simulink model "Steam_Turbine"  (R2024b)
settings: Solver=VariableStepAuto  StartTime=0.0  StopTime=50  RelTol=1e-3
settings Model: Creator=HP  LastModifiedBy=HP

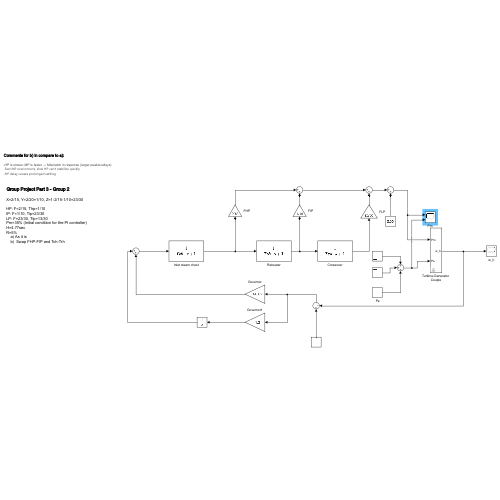
[thumbnail: Simulink's stored preview of the top-level diagram]
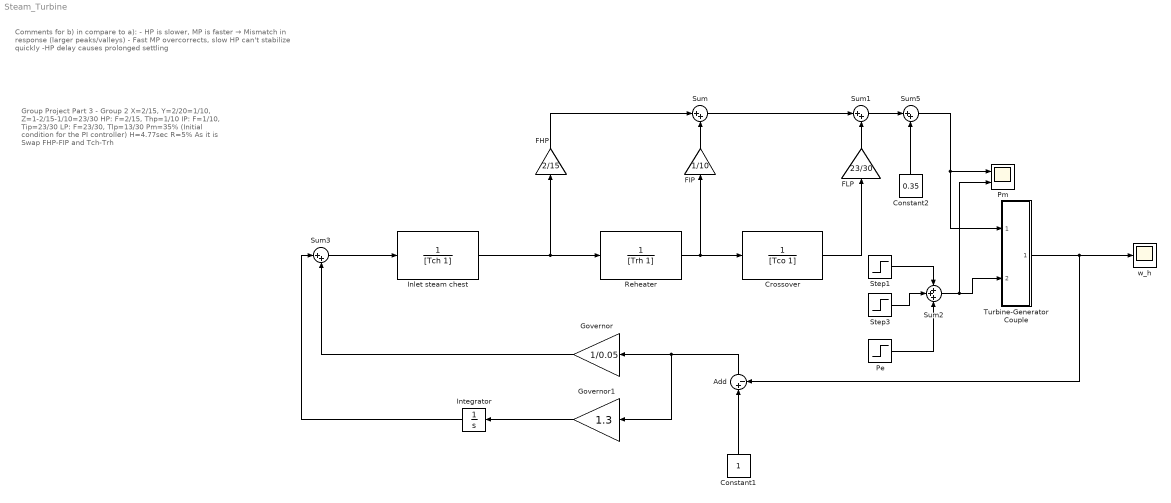
== system Steam_Turbine ==
  note: Comments for b) in compare to a):
      |
      | - HP is slower, MP is faster → Mismatch in response (larger peaks/valleys)
      | - Fast MP overcorrects, slow HP can't stabilize quickly
      | -HP delay causes prolonged settling
  note: Group Project Part 3 - Group 2
      |
      | X=2/15, Y=2/20=1/10, Z=1-2/15-1/10=23/30
      |
      | HP: F=2/15, Thp=1/10
      | IP: F=1/10, Tip=23/30
      | LP: F=23/30, Tlp=13/30
      | Pm=35% (Initial condition for the PI controller)
      | H=4.77sec
      | R=5%
      | As it is
      | Swap FHP-FIP and Tch-Trh
  " Pe" : Step  Time=15  Before=0.15  After=0.45  SampleTime=0
  Add : Sum  Inputs=|+-
  Constant1 : Constant
  Constant2 : Constant  Value=0.35
  Crossover : TransferFcn  Denominator=[Tco 1]  mask{Tco=13/30}
      mask prompts: Tco "Crossover Time Constant / Low-Pressure (LP) Turbine Time Constant)"
      mask DialogControl ParameterGroupVar Prompt: Parameters
  FHP : Gain  Gain=2/15
  FIP : Gain  Gain=1/10
  FLP : Gain  Gain=23/30
  Governor : Gain  Gain=1/0.05
  Governor1 : Gain  Gain=1.3
  Inlet steam chest : TransferFcn  Denominator=[Tch 1]  mask{Tch=1/10}
      mask prompts: Tch "HP cynlinder time constant"
      mask DialogControl ParameterGroupVar Prompt: Parameters
  Integrator : Integrator
  Pm : Scope  NumInputPorts=2
  Reheater : TransferFcn  Denominator=[Trh 1]  mask{Trh=23/30}
      mask prompts: Trh "Reheater Time Constant"
      mask DialogControl ParameterGroupVar Prompt: Parameters
  Step1 : Step  Time=5  Before=0.10  After=0.35  SampleTime=0
  Step3 : Step  Time=10  Before=0.10  After=-0.30  SampleTime=0
  Sum{,1,3,5} (4 alike) : Sum  Inputs=|++
  Sum2 : Sum  Inputs=+++
  Turbine-Generator Couple : Subsystem  mask{Hh=4.77, w_ini=1}
      mask prompts: Hh "H/E Inertia Constant"; w_ini "Initial omega"
  w_h : Scope
  wires:
  Sum5/1 -> Turbine-Generator Couple/1(Pm), Pm/1
  Inlet steam chest/1 -> FHP/1, Reheater/1
  FHP/1 -> Sum/1
  Sum/1 -> Sum1/1
  FLP/1 -> Sum1/2
  FIP/1 -> Sum/2
  Turbine-Generator Couple/1(w_h) -> Add/2, w_h/1
  Constant1/1 -> Add/1
  Add/1 -> Governor1/1, Governor/1
  Reheater/1 -> Crossover/1, FIP/1
  Crossover/1 -> FLP/1
  Governor1/1 -> Integrator/1
  Integrator/1 -> Sum3/1
  Governor/1 -> Sum3/2
  Sum3/1 -> Inlet steam chest/1
  Step1/1 -> Sum2/1
  " Pe"/1 -> Sum2/3
  Step3/1 -> Sum2/2
  Sum2/1 -> Pm/2, Turbine-Generator Couple/2(Pe)
  Sum1/1 -> Sum5/1
  Constant2/1 -> Sum5/2

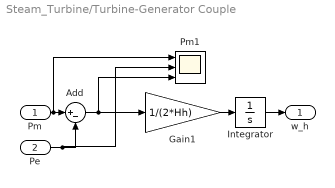
== system Steam_Turbine/Turbine-Generator Couple ==
  Pm : Inport
  Pe : Inport  Port=2
  Add : Sum  Inputs=|+-
  Gain1 : Gain  Gain=1/(2*Hh)
  Integrator : Integrator  InitialCondition=w_ini
  Pm1 : Scope  NumInputPorts=3
  w_h : Outport
  wires:
  Pm/1 -> Pm1/1, Add/1
  Gain1/1 -> Integrator/1
  Integrator/1 -> w_h/1
  Pe/1 -> Pm1/2, Add/2
  Add/1 -> Pm1/3, Gain1/1
